simulink model "Example_1"  (Simulink 7.6)
settings: Solver=ode45  StartTime=0.0  StopTime=10.0  RelTol=1e-3
libraries: utility x1
settings Model: Creator=Ivan  LastModifiedBy=Ivan

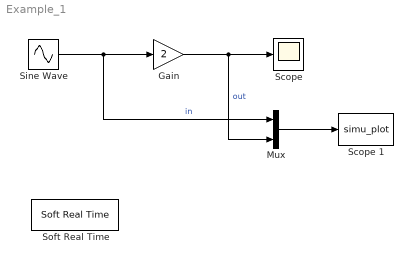
== system Example_1 ==
  Gain : Gain  Gain=2
  Mux : Mux  Inputs=2
  Scope : Scope
  Scope 1 : M-S-Function  FunctionName=simu_plot  Parameters=decim, T_refresh  mask{decim=1, T_refresh=2}
      mask prompts: decim "Decimation"; T_refresh "Redraw time"
      settings: DeleteFcn=simu_figure('delete',gcbh)  NameChangeFcn=simu_figure('namechange',gcbh)  DestroyFcn=simu_figure('destroy',gcbh)  OpenFcn=simu_figure('open',gcbh)  CloseFcn=simu_figure('close',gcbh)  ParentCloseFcn=simu_figure('parentclose',gcbh)
      mask Display: disp('Simu-plot');
  Sine Wave : Sin  SampleTime=0
  Soft Real Time : utility/Soft Real Time  x=1  enabled=1
  wires:
  Sine Wave/1 -> Gain/1, Mux/1  "in"
  Gain/1 -> Scope/1, Mux/2  "out"
  Mux/1 -> Scope 1/1
